simulink model "CombinedPIDFuzz"  (R2016a)
settings: Solver=VariableStepAuto  StartTime=0.0  StopTime=10.0  RelTol=1e-3
values from neighbouring files (symbols this model uses):
  Bm = 0.002953    [April2code.mat]    (also in April6code.mat)
  Jm = 0.02215    [April2code.mat]    (also in April6code.mat)
  Kb = 1.28    [April2code.mat]    (also in April6code.mat)
  Kd = 0.45    [April2code.mat]    (also in April6code.mat = 0.7)
  Kp = 5    [April2code.mat]    (also in April6code.mat = 8)
  Kt = 1.28    [April2code.mat]    (also in April6code.mat)
  La = 0.1215    [April2code.mat]    (also in April6code.mat)
  Ra = 11.2    [April2code.mat]    (also in April6code.mat)
libraries: checkpacklib x1, fuzblock x1
settings Model: Creator=Dheeraj Singh  LastModifiedBy=Dheeraj Singh

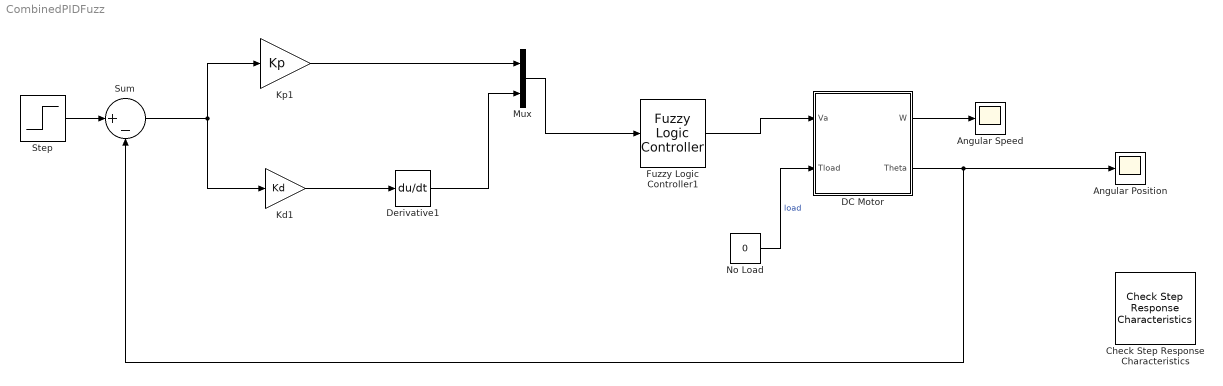
== system CombinedPIDFuzz ==
  Angular Position : Scope
  Angular Speed : Scope
  Check Step Response Characteristics : checkpacklib/Check Step Response  Characteristics  InstantiateOnLoad=on  enabled=on  stopWhenAssertionFail=off  export=off  ViewDlgPos=[]  OpenViewOnLoad=off  LaunchViewOnOpen=off  TimeUnits=seconds  EnableStepResponseBound=on  InitialValue=0  FinalValue=1  StepTime=0  RiseTime=5  PercentRise=80  SettlingTime=7  PercentSettling=1  PercentOvershoot=10  PercentUndershoot=1
  DC Motor : Subsystem
  Derivative1 : Derivative  CoefficientInTFapproximation=1
  Fuzzy Logic Controller1 : fuzblock/Fuzzy Logic  Controller  fis=FuzData
  Kd1 : Gain  Gain=Kd
  Kp1 : Gain  Gain=Kp
  Mux : Mux  Inputs=2
  No Load : Constant  Value=0
  Step : Step  SampleTime=0
  Sum : Sum  Inputs=|+-
  wires:
  No Load/1 -> DC Motor/2(Tload)  "load"
  DC Motor/1(W) -> Angular Speed/1
  Step/1 -> Sum/1
  Kd1/1 -> Derivative1/1
  Kp1/1 -> Mux/1
  Derivative1/1 -> Mux/2
  Fuzzy Logic Controller1/1 -> DC Motor/1(Va)
  Mux/1 -> Fuzzy Logic Controller1/1
  Sum/1 -> Kp1/1, Kd1/1
  DC Motor/2(Theta) -> Sum/2, Angular Position/1

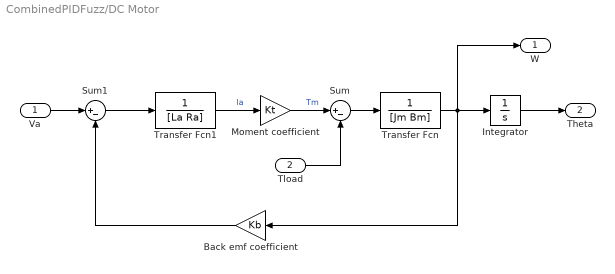
== system CombinedPIDFuzz/DC Motor ==
  Va : Inport
  Tload : Inport  Port=2
  Back emf coefficient : Gain  Gain=Kb
  Integrator : Integrator
  Moment coefficient : Gain  Gain=Kt
  Sum : Sum  Inputs=|+-
  Sum1 : Sum  Inputs=|+-
  Transfer Fcn : TransferFcn  Denominator=[Jm Bm]
  Transfer Fcn1 : TransferFcn  Denominator=[La Ra]
  W : Outport
  Theta : Outport  Port=2
  wires:
  Transfer Fcn1/1 -> Moment coefficient/1  "la"
  Sum/1 -> Transfer Fcn/1
  Va/1 -> Sum1/1
  Moment coefficient/1 -> Sum/1  "Tm"
  Transfer Fcn/1 -> W/1, Back emf coefficient/1, Integrator/1
  Integrator/1 -> Theta/1
  Tload/1 -> Sum/2
  Sum1/1 -> Transfer Fcn1/1
  Back emf coefficient/1 -> Sum1/2
